simulink model "it2_only"  (R2023a)
settings: Solver=VariableStepAuto  StartTime=0.0  StopTime=10.0  RelTol=1e-3
libraries: fuzblock x1
settings Model: Creator=yingb  LastModifiedBy=yingb

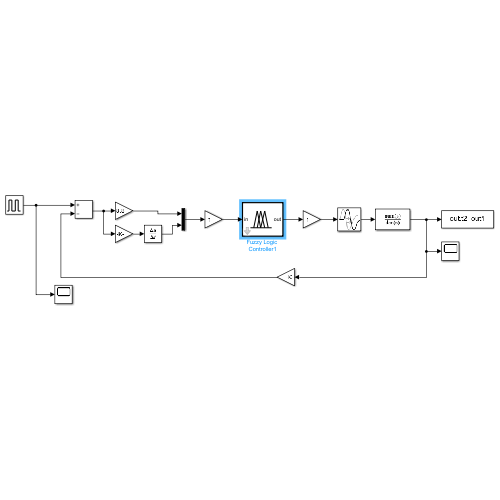
[thumbnail: Simulink's stored preview of the top-level diagram]
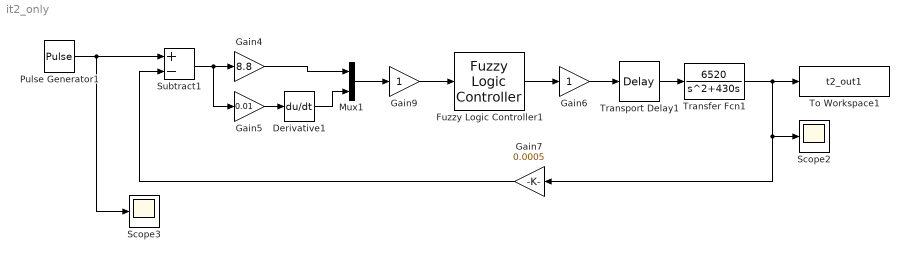
== system it2_only ==
  Derivative1 : Derivative
  Fuzzy Logic Controller1 : fuzblock/Fuzzy Logic  Controller  FIS='itype2_fis.fis'  OutputSampleNumber=101  DataType=double  FuzzifiedInputs=off  RuleFiringStrengths=off  RuleOutputs=off  AggregatedOutputs=off  SimulateUsing=Interpreted execution  OutOfRangeInputValueMessage=warning  NoRuleFiredMessage=warning  EmptyOutputFuzzySetMessage=warning
  Gain4 : Gain  Gain=8.8
  Gain5 : Gain  Gain=0.01  OutMin=[-0.15]  OutMax=[0.15]
  Gain6 : Gain
  Gain7 : Gain  Gain=0.0005
  Gain9 : Gain
  Mux1 : Mux  Inputs=2
  Pulse Generator1 : DiscretePulseGenerator  PulseType=Time based  Amplitude=0.3  Period=4  PulseWidth=50
  Scope2 : Scope
      settings: Tag=t1_fis
  Scope3 : Scope
      settings: Tag=t1_fis
  Subtract1 : Sum  Inputs=+-
  To Workspace1 : ToWorkspace  VariableName=t2_out1  SaveFormat=Timeseries  SampleTime=0.005
  Transfer Fcn1 : TransferFcn  Numerator=[6520]  Denominator=[1 430 0]  ParameterTunability=Optimized
  Transport Delay1 : TransportDelay  DelayTime=0.005
  wires:
  Derivative1/1 -> Mux1/2
  Mux1/1 -> Gain9/1
  Pulse Generator1/1 -> Scope3/1, Subtract1/1
  Gain9/1 -> Fuzzy Logic Controller1/1
  Gain4/1 -> Mux1/1
  Transfer Fcn1/1 -> Scope2/1, Gain7/1, To Workspace1/1
  Gain6/1 -> Transport Delay1/1
  Transport Delay1/1 -> Transfer Fcn1/1
  Gain5/1 -> Derivative1/1
  Fuzzy Logic Controller1/1 -> Gain6/1
  Gain7/1 -> Subtract1/2
  Subtract1/1 -> Gain5/1, Gain4/1
